simulink model "power_machines_Hatch"  (R2014a)
settings: Solver=ode23tb  SolverMode=SingleTasking  StartTime=0.0  StopTime=60  RelTol=1e-4
undefined symbols (not defined in the file or in its folder): A, B, C, Continuous, Dd, Ka, Ke, Kf, SeVe1, SeVe2, spsAC1AModel, Ta, Te, Tf, VAmax, VAmin, Ve0, Ve1, Ve2, Vfe0, VRmax, VRmin
undefined symbols (not defined in the file): Tb, Tc
libraries: sps_avr x19, powerlib x16, simulink_extras x4
(part 1 of 2)
Description:
  | Copyright 2008-2014 The MathWorks, Inc.
settings Model: FPTRunName=Active  ExtModeTrigMode=oneshot  ExtModeArmWhenConnect=off  ExtModeAutoUpdateStatusClock=off  Creator=MathWorks  LastModifiedBy=jdlara
settings SolverCC: ZeroCrossAlgorithm=Adaptive
settings DataIOCC: LimitDataPoints=off  SignalLoggingSaveFormat=ModelDataLogs  SignalLoggingName=sigsOut  OutputTimes=[0:1/20:10]
settings OptimizationCC: BlockReduction=off  BooleanDataType=off  ExpressionDepthLimit=2147483647  InitFltsAndDblsToZero=on  EfficientMapNaN2IntZero=off
settings DebuggingCC: UnderspecifiedInitializationDetection=Classic  CheckExecutionContextPreStartOutputMsg=on  CheckExecutionContextRuntimeOutputMsg=on  SignalResolutionControl=TryResolveAllWithWarning  IgnoredZcDiagnostic=none  SolverPrmCheckMsg=none  MultiTaskDSMMsg=warning  MultiTaskCondExecSysMsg=none  SigSpecEnsureSampleTimeMsg=none  FcnCallInpInsideContextMsg=UseLocalSettings  UnconnectedInputMsg=none  UnconnectedOutputMsg=none  UnconnectedLineMsg=none  StateNameClashWarn=warning
settings HardwareCC: ProdHWDeviceType=Specified  TargetUnknown=on
settings RTWCC: IncludeERTFirstTime=on
settings CodeAppCC: IgnoreCustomStorageClasses=off
settings GRTTargetCC: TargetFcnLib=ansi_tfl_tmw.mat  CombineOutputUpdateFcns=off  GRTInterface=on

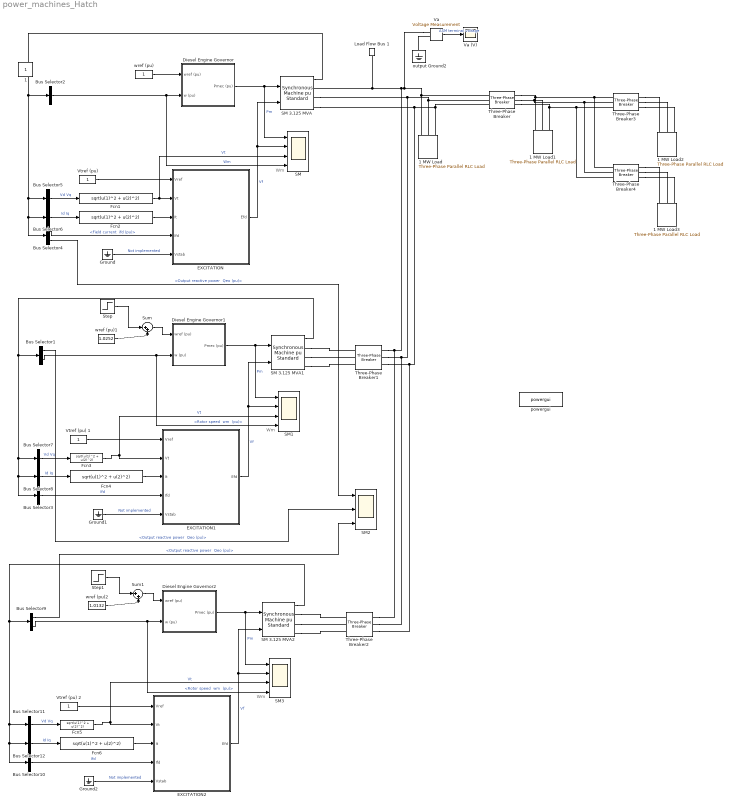
== system power_machines_Hatch ==
  note: Wm
  note: Wm
  note: Wm
  1 MW Load : powerlib/Elements/Three-Phase Parallel RLC Load  LConnTagsString=A|B|C  Configuration=Y (grounded)  NominalVoltage=2400  NominalFrequency=60  ActivePower=2.8e+006  InductivePower=8e5  CapacitivePower=0  Measurements=None  LoadType=constant Z
  1 MW Load1 : powerlib/Elements/Three-Phase Parallel RLC Load  LConnTagsString=A|B|C  Configuration=Y (grounded)  NominalVoltage=2400  NominalFrequency=60  ActivePower=1.5e+006  InductivePower=8e5  CapacitivePower=0  Measurements=None  LoadType=constant Z
  1 MW Load2 : powerlib/Elements/Three-Phase Parallel RLC Load  LConnTagsString=A|B|C  Configuration=Y (grounded)  NominalVoltage=2400  NominalFrequency=60  ActivePower=1.0e+006  InductivePower=8e5  CapacitivePower=0  Measurements=None  LoadType=constant Z
  1 MW Load3 : powerlib/Elements/Three-Phase Parallel RLC Load  LConnTagsString=A|B|C  Configuration=Y (grounded)  NominalVoltage=2400  NominalFrequency=60  ActivePower=1.1e+006  InductivePower=8e4  CapacitivePower=0  Measurements=None  LoadType=constant Z
  Bus Selector1 : BusSelector  OutputSignals="Output reactive power  Qeo (pu),Mechanical.Rotor speed  wm  (pu)"
  Bus Selector10 : BusSelector  OutputSignals="dq0 components.Field current  ifd (pu)"  OutputAsBus=on
  Bus Selector11 : BusSelector  OutputSignals="dq0 components.Stator voltage  vd (pu),dq0 components.Stator voltage  vq (pu)"  OutputAsBus=on
  Bus Selector12 : BusSelector  OutputSignals="dq0 components.Stator current  id (pu),dq0 components.Stator current  iq (pu)"  OutputAsBus=on
  Bus Selector2 : BusSelector  OutputSignals="Mechanical.Rotor speed  wm  (pu)"  OutputAsBus=on
  Bus Selector3 : BusSelector  OutputSignals="dq0 components.Field current  ifd (pu)"  OutputAsBus=on
  Bus Selector4 : BusSelector  OutputSignals="dq0 components.Field current  ifd (pu),Output reactive power  Qeo (pu)"
  Bus Selector5 : BusSelector  OutputSignals="dq0 components.Stator voltage  vd (pu),dq0 components.Stator voltage  vq (pu)"  OutputAsBus=on
  Bus Selector6 : BusSelector  OutputSignals="dq0 components.Stator current  id (pu),dq0 components.Stator current  iq (pu)"  OutputAsBus=on
  Bus Selector7 : BusSelector  OutputSignals="dq0 components.Stator voltage  vd (pu),dq0 components.Stator voltage  vq (pu)"  OutputAsBus=on
  Bus Selector8 : BusSelector  OutputSignals="dq0 components.Stator current  id (pu),dq0 components.Stator current  iq (pu)"  OutputAsBus=on
  Bus Selector9 : BusSelector  OutputSignals="Output reactive power  Qeo (pu),Mechanical.Rotor speed  wm  (pu)"
  Diesel Engine Governor : Subsystem  mask(Diesel Engine & Governor){K=40, Tr=[0.01 0.02 0.2], Ta=[0.25 0.009 0.0384], Tlim=[0 1.1], Td=0.024, Pm0=0.30302}
      mask prompts: K "Regulator gain K:"; Tr "Regulator time constants [T1 T2 T3 ] (s) :"; Ta "Actuator time constants [T4 T5 T6] (s) :"; Tlim "Torque limits [Tmin Tmax] (pu) :"; Td "Engine time delay Td (s) :"; Pm0 "Initial value of mechanical power  Pm0 (pu) :"
      mask help:
      | This block implements a diesel engine and governor system:
      | 1st and 2nd inputs: Desired and actual speed (pu)
      | Output: Diesel engine mechanical power.Motor inertia should be combined with generator.
      | Controller transfer function:
      |      Hc=K.(1+T3.s)/(1+T1.s+T1.T2.s^2)
      | Actuator transfer function :
      |      Ha= (1+T4.s) / [ (s (1+T5.s)(1+T6.s) ]
      | Motor :
      |      Time delay Td
      |
      | (See reference in Tutorial Session 5)
  Diesel Engine Governor1 : Subsystem  mask(Diesel Engine & Governor){K=40, Tr=[0.012 0.02 0.2], Ta=[0.25 0.009 0.0384], Tlim=[0 1.1], Td=0.024, Pm0=0.70051}
      mask prompts: K "Regulator gain K:"; Tr "Regulator time constants [T1 T2 T3 ] (s) :"; Ta "Actuator time constants [T4 T5 T6] (s) :"; Tlim "Torque limits [Tmin Tmax] (pu) :"; Td "Engine time delay Td (s) :"; Pm0 "Initial value of mechanical power  Pm0 (pu) :"
      mask help:
      | This block implements a diesel engine and governor system:
      | 1st and 2nd inputs: Desired and actual speed (pu)
      | Output: Diesel engine mechanical power.Motor inertia should be combined with generator.
      | Controller transfer function:
      |      Hc=K.(1+T3.s)/(1+T1.s+T1.T2.s^2)
      | Actuator transfer function :
      |      Ha= (1+T4.s) / [ (s (1+T5.s)(1+T6.s) ]
      | Motor :
      |      Time delay Td
      |
      | (See reference in Tutorial Session 5)
  Diesel Engine Governor2 : Subsystem  mask(Diesel Engine & Governor){K=40, Tr=[0.012 0.02 0.2], Ta=[0.25 0.009 0.0384], Tlim=[0 1.1], Td=0.024, Pm0=0.70051}
      mask prompts: K "Regulator gain K:"; Tr "Regulator time constants [T1 T2 T3 ] (s) :"; Ta "Actuator time constants [T4 T5 T6] (s) :"; Tlim "Torque limits [Tmin Tmax] (pu) :"; Td "Engine time delay Td (s) :"; Pm0 "Initial value of mechanical power  Pm0 (pu) :"
      mask help:
      | This block implements a diesel engine and governor system:
      | 1st and 2nd inputs: Desired and actual speed (pu)
      | Output: Diesel engine mechanical power.Motor inertia should be combined with generator.
      | Controller transfer function:
      |      Hc=K.(1+T3.s)/(1+T1.s+T1.T2.s^2)
      | Actuator transfer function :
      |      Ha= (1+T4.s) / [ (s (1+T5.s)(1+T6.s) ]
      | Motor :
      |      Time delay Td
      |
      | (See reference in Tutorial Session 5)
  EXCITATION : Subsystem  Variant=on  OverrideUsingVariant=Variant1
      settings: AttributesFormatString=%<BlockChoice>
  EXCITATION1 : Subsystem  Variant=on  OverrideUsingVariant=Variant1
      settings: AttributesFormatString=%<BlockChoice>
  EXCITATION2 : Subsystem  Variant=on  OverrideUsingVariant=Variant1
      settings: AttributesFormatString=%<BlockChoice>
  Fcn{1..6} (6 alike) : Fcn  Expr=sqrt(u(1)^2 + u(2)^2)
  Ground : Ground
  Ground1 : Ground
  Ground2 : Ground
  Load Flow Bus 1 : powerlib/Measurements/Load Flow Bus  LConnTagsString=a  ID=B2  Vbase=2.4e3  Vref=1  Vangle=0  VLF=1  angleLF=0
      settings: AttributesFormatString=%<ID>\n%<Vbase>V\n%<VLF>pu\n%<angleLF>deg.
  SM : Scope  NumInputPorts=4
      settings: TimeRange=45  YMin=0.3~-5~0~0.96  YMax=0.7000000000000001~10~1.5~1.04  SaveName=Pmec_SM1  DataFormat=Structure  Decimation=10
  SM 3.125 MVA : powerlib/Machines/Synchronous Machine pu Standard  PresetModel=No  MechanicalLoad=Mechanical power Pm  ShowDetailedParameters=on  RotorType=Salient-pole  Units=per unit standard parameters  MeasurementBus=off  NominalParameters="[ 3.125e6  2400  60]"  Reactances1=[ 31 32 33 34 35 36 37 ]  Reactances2=[ 1.56, 0.296, 0.177, 1.06, 0.177, 0.052 ]  dAxisTimeConstants=Short-circuit  qAxisTimeConstants=Open-circuit  TimeConstants1=[]  TimeConstants2=[]  TimeConstants3=[]  TimeConstants4=[]  TimeConstants5=[ 3.7, 0.05, 0.05 ]  TimeConstants6=[ 8.0, 0.03, 0.3371, 0.0295 ]  TimeConstants7=[0.024 0.006 0.006]  TimeConstants8=[]  StatorResistance=0.0036  Mechanical="[ 1.07  0 2]"  PolePairs=2  InitialConditions=[0 -78.3178 0.589753 0.589753 0.589753 -59.2242 -179.224 60.7758 1.84938]  SetSaturation=off  Saturation=[0.211 0.418 1.0 1.25 1.72 3.35 ;0.25 0.50 1.0 1.1 1.2 1.4]  LoadFlowParameters=[2 0 0 0]  TsPowergui=0  TsBlock=-1  IterativeModel=Forward Euler  BusType=swing  Pref=0  Qref=0  Qmin=-Inf  Qmax=Inf  PLF=0  QLF=0
      settings: AttributesFormatString=\n\n
  SM 3.125 MVA1 : powerlib/Machines/Synchronous Machine pu Standard  PresetModel=No  MechanicalLoad=Mechanical power Pm  ShowDetailedParameters=on  RotorType=Salient-pole  Units=per unit standard parameters  MeasurementBus=off  NominalParameters="[ 3.125e6  2400  60]"  Reactances1=[ 31 32 33 34 35 36 37 ]  Reactances2=[ 1.56, 0.296, 0.177, 1.06, 0.177, 0.052 ]  dAxisTimeConstants=Short-circuit  qAxisTimeConstants=Open-circuit  TimeConstants1=[]  TimeConstants2=[]  TimeConstants3=[]  TimeConstants4=[]  TimeConstants5=[ 3.7, 0.05, 0.05 ]  TimeConstants6=[ 8.0, 0.03, 0.3371, 0.0295 ]  TimeConstants7=[0.024 0.006 0.006]  TimeConstants8=[]  StatorResistance=0.0036  Mechanical="[ 1.07  0 2]"  PolePairs=2  InitialConditions=[0 -57.177 0.707662 0.707662 0.707662 -10.4209 -130.421 109.579 1.60133]  SetSaturation=off  Saturation=[0.211 0.418 1.0 1.25 1.72 3.35 ;0.25 0.50 1.0 1.1 1.2 1.4]  LoadFlowParameters=[4 0 0 0]  TsPowergui=0  TsBlock=-1  IterativeModel=Forward Euler  BusType=PQ  Pref=0.6987068134*3.125e6  Qref=0.4e6  Qmin=-Inf  Qmax=Inf  PLF=0  QLF=0
      settings: AttributesFormatString=\n\n
  SM 3.125 MVA2 : powerlib/Machines/Synchronous Machine pu Standard  PresetModel=No  MechanicalLoad=Mechanical power Pm  ShowDetailedParameters=on  RotorType=Salient-pole  Units=per unit standard parameters  MeasurementBus=off  NominalParameters="[ 3.125e6  2400  60]"  Reactances1=[ 31 32 33 34 35 36 37 ]  Reactances2=[ 1.56, 0.296, 0.177, 1.06, 0.177, 0.052 ]  dAxisTimeConstants=Short-circuit  qAxisTimeConstants=Open-circuit  TimeConstants1=[]  TimeConstants2=[]  TimeConstants3=[]  TimeConstants4=[]  TimeConstants5=[ 3.7, 0.05, 0.05 ]  TimeConstants6=[ 8.0, 0.03, 0.3371, 0.0295 ]  TimeConstants7=[0.024 0.006 0.006]  TimeConstants8=[]  StatorResistance=0.0036  Mechanical="[ 1.07  0 2]"  PolePairs=2  InitialConditions=[0 -57.177 0.707662 0.707662 0.707662 -10.4209 -130.421 109.579 1.60133]  SetSaturation=off  Saturation=[0.211 0.418 1.0 1.25 1.72 3.35 ;0.25 0.50 1.0 1.1 1.2 1.4]  LoadFlowParameters=[4 0 0 0]  TsPowergui=0  TsBlock=-1  IterativeModel=Forward Euler  BusType=PQ  Pref=0.6987068134*3.125e6  Qref=0.4e6  Qmin=-Inf  Qmax=Inf  PLF=0  QLF=0
      settings: AttributesFormatString=\n\n
  SM1 : Scope  NumInputPorts=4
      settings: TimeRange=4.8  YMin=0.7117940298507462~-5~1.0006~0.950028  YMax=0.7165940298507462~10~1.0016~1.05003  SaveName=Pmec_SM  DataFormat=Structure  Decimation=10
  SM2 : Scope  NumInputPorts=3
      settings: TimeRange=10  YMin=0~0~-5  YMax=1~1~5  SaveName=Pmec_SM2  DataFormat=Structure  Decimation=10
  SM3 : Scope  NumInputPorts=4
      settings: TimeRange=4.8  YMin=0.7117940298507462~-5~1.0006~0.950028  YMax=0.7165940298507462~10~1.0016~1.05003  SaveName=Pmec_SM3  DataFormat=Structure  Decimation=10
  Step : Step  Time=20  After=0.008  SampleTime=0
  Step1 : Step  Time=10  After=0.008  SampleTime=0
  Sum : Sum  Inputs=|++
  Sum1 : Sum  Inputs=|++
  Three-Phase Breaker : powerlib/Elements/Three-Phase Breaker  InitialState=closed  SwitchA=on  SwitchB=on  SwitchC=on  SwitchTimes="[92  170]"  External=off  BreakerResistance=0.01  SnubberResistance=1e6  SnubberCapacitance=inf  Measurements=None
  Three-Phase Breaker1 : powerlib/Elements/Three-Phase Breaker  InitialState=closed  SwitchA=on  SwitchB=on  SwitchC=on  SwitchTimes="[120  170]"  External=off  BreakerResistance=0.01  SnubberResistance=1e6  SnubberCapacitance=inf  Measurements=None
  Three-Phase Breaker2 : powerlib/Elements/Three-Phase Breaker  InitialState=closed  SwitchA=on  SwitchB=on  SwitchC=on  SwitchTimes="[120  170]"  External=off  BreakerResistance=0.01  SnubberResistance=1e6  SnubberCapacitance=inf  Measurements=None
  Three-Phase Breaker3 : powerlib/Elements/Three-Phase Breaker  InitialState=closed  SwitchA=on  SwitchB=on  SwitchC=on  SwitchTimes=[30 70]  External=off  BreakerResistance=0.01  SnubberResistance=1e6  SnubberCapacitance=inf  Measurements=None
  Three-Phase Breaker4 : powerlib/Elements/Three-Phase Breaker  InitialState=open  SwitchA=on  SwitchB=on  SwitchC=on  SwitchTimes=[40 70]  External=off  BreakerResistance=0.01  SnubberResistance=1e6  SnubberCapacitance=inf  Measurements=None
  Va : powerlib/Measurements/Voltage Measurement  Tag=PoWeRsYsTeMmEaSuReMeNt  PhasorSimulation=off  OutputType=Magnitude  PSBequivalent=0
  Va (V) : Scope
      settings: TickLabels=on  TimeRange=5  YMin=-3000  YMax=3000
  "Vtref (pu) " : Constant
  Vtref (pu) 1 : Constant
  Vtref (pu) 2 : Constant
  output Ground2 : powerlib/Elements/Ground  LConnTagsString=a
  powergui : powerlib/powergui  Priority=2  SimulationMode=Continuous  SolverType=Tustin  SampleTime=50e-6  frequency=60  SPID=off  DisableSnubberDevices=off  DisableRonSwitches=off  DisableVfSwitches=off  SwTol=0  Interpol=off  DisplayEquations=off  Ts=0  methode=off  frequencyindice=60  Pbase=1e6  ErrMax=0.0001  Iterations=50  UnitsV=kV  UnitsW=MW  FunctionMessages=off  echomessages=off  HookPort=off  EnableUseOfTLC=off  x0status=blocks  RestoreLinks=warning  ResistiveCurrentMeasurement=off  Frange=logspace(0,3,50)  Ylog=off  Xlog=off  ShowGrid=off  save=off  variable=ZData  structure=0  ZoomFFT=on  StartTime=0.0  cycles=2  DisplayStyle=off  fundamental=60  FreqAxis=off  MaxFrequency=1000  frequencyindicesteady=1  RmsSteady=1  display=off
  wref (pu) : Constant
  wref (pu)1 : Constant  Value=1.0252
  wref (pu)2 : Constant  Value=1.0132
  1 : Constant  IOType=siggen
  wires:
  Va/1 -> Va (V)/1  "ASM terminal voltage"
  Diesel Engine Governor/1(Pmec (pu)) -> SM/1, SM 3.125 MVA/1  "Pm"
  Fcn2/1 -> EXCITATION/3(It)
  Bus Selector4/1 -> EXCITATION/4(Ifd)  "<Field current  ifd (pu)>"
  Bus Selector6/1 -> Fcn2/1  "Id Iq"
  Ground/1 -> EXCITATION/5(Vstab)  "Not implemented"
  Bus Selector5/1 -> Fcn1/1  "Vd Vq"
  Bus Selector2/1 -> Diesel Engine Governor/2(w (pu)), SM/4  "Wm"
  Fcn1/1 -> EXCITATION/2(Vt), SM/3  "Vt"
  EXCITATION/1(Efd) -> SM 3.125 MVA/2, SM/2  "Vf"
  "Vtref (pu) "/1 -> EXCITATION/1(Vref)
  wref (pu)/1 -> Diesel Engine Governor/1(wref (pu))
  SM 3.125 MVA/1 -> Bus Selector2/1, Bus Selector5/1, Bus Selector6/1, Bus Selector4/1
  Diesel Engine Governor1/1(Pmec (pu)) -> SM1/1, SM 3.125 MVA1/1  "Pm"
  Fcn4/1 -> EXCITATION1/3(It)
  Bus Selector3/1 -> EXCITATION1/4(Ifd)  "Ifd"
  Bus Selector8/1 -> Fcn4/1  "Id Iq"
  Ground1/1 -> EXCITATION1/5(Vstab)  "Not implemented"
  Bus Selector7/1 -> Fcn3/1  "Vd Vq"
  Bus Selector1/2 -> Diesel Engine Governor1/2(w (pu)), SM1/4  "<Rotor speed  wm  (pu)>"
  Fcn3/1 -> EXCITATION1/2(Vt), SM1/3  "Vt"
  EXCITATION1/1(Efd) -> SM1/2, SM 3.125 MVA1/2  "Vf"
  Vtref (pu) 1/1 -> EXCITATION1/1(Vref)
  SM 3.125 MVA1/1 -> Bus Selector1/1, Bus Selector7/1, Bus Selector8/1, Bus Selector3/1
  Step/1 -> Sum/1
  wref (pu)1/1 -> Sum/2
  Sum/1 -> Diesel Engine Governor1/1(wref (pu))
  Bus Selector4/2 -> SM2/1  "<Output reactive power  Qeo (pu)>"
  Bus Selector1/1 -> SM2/2  "<Output reactive power  Qeo (pu)>"
  Diesel Engine Governor2/1(Pmec (pu)) -> SM3/1, SM 3.125 MVA2/1  "Pm"
  Fcn6/1 -> EXCITATION2/3(It)
  Bus Selector10/1 -> EXCITATION2/4(Ifd)  "Ifd"
  Bus Selector12/1 -> Fcn6/1  "Id Iq"
  Ground2/1 -> EXCITATION2/5(Vstab)  "Not implemented"
  Bus Selector11/1 -> Fcn5/1  "Vd Vq"
  Bus Selector9/2 -> Diesel Engine Governor2/2(w (pu)), SM3/4  "<Rotor speed  wm  (pu)>"
  Fcn5/1 -> EXCITATION2/2(Vt), SM3/3  "Vt"
  EXCITATION2/1(Efd) -> SM3/2, SM 3.125 MVA2/2  "Vf"
  Vtref (pu) 2/1 -> EXCITATION2/1(Vref)
  SM 3.125 MVA2/1 -> Bus Selector9/1, Bus Selector11/1, Bus Selector12/1, Bus Selector10/1
  Step1/1 -> Sum1/1
  wref (pu)2/1 -> Sum1/2
  Sum1/1 -> Diesel Engine Governor2/1(wref (pu))
  Bus Selector9/1 -> SM2/3  "<Output reactive power  Qeo (pu)>"
  connections:
  output Ground2/LConn1 -- Va/LConn2
  SM 3.125 MVA/RConn2 -- Three-Phase Breaker2/RConn2 -- Three-Phase Breaker1/RConn2 -- Three-Phase Breaker/LConn2 -- 1 MW Load/LConn2
  Va/LConn1 -- Three-Phase Breaker2/RConn1 -- Three-Phase Breaker1/RConn1 -- SM 3.125 MVA/RConn1 -- Load Flow Bus 1/LConn1 -- Three-Phase Breaker/LConn1 -- 1 MW Load/LConn1
  SM 3.125 MVA/RConn3 -- Three-Phase Breaker2/RConn3 -- Three-Phase Breaker1/RConn3 -- 1 MW Load/LConn3 -- Three-Phase Breaker/LConn3
  Three-Phase Breaker/RConn1 -- Three-Phase Breaker4/LConn1 -- Three-Phase Breaker3/LConn1 -- 1 MW Load1/LConn1
  Three-Phase Breaker/RConn2 -- Three-Phase Breaker4/LConn2 -- Three-Phase Breaker3/LConn2 -- 1 MW Load1/LConn2
  Three-Phase Breaker/RConn3 -- Three-Phase Breaker4/LConn3 -- Three-Phase Breaker3/LConn3 -- 1 MW Load1/LConn3
  SM 3.125 MVA1/RConn1 -- Three-Phase Breaker1/LConn1
  SM 3.125 MVA1/RConn2 -- Three-Phase Breaker1/LConn2
  SM 3.125 MVA1/RConn3 -- Three-Phase Breaker1/LConn3
  SM 3.125 MVA2/RConn1 -- Three-Phase Breaker2/LConn1
  SM 3.125 MVA2/RConn3 -- Three-Phase Breaker2/LConn3
  SM 3.125 MVA2/RConn2 -- Three-Phase Breaker2/LConn2
  Three-Phase Breaker3/RConn2 -- 1 MW Load2/LConn2
  Three-Phase Breaker3/RConn1 -- 1 MW Load2/LConn1
  Three-Phase Breaker3/RConn3 -- 1 MW Load2/LConn3
  Three-Phase Breaker4/RConn3 -- 1 MW Load3/LConn3
  Three-Phase Breaker4/RConn1 -- 1 MW Load3/LConn1
  Three-Phase Breaker4/RConn2 -- 1 MW Load3/LConn2

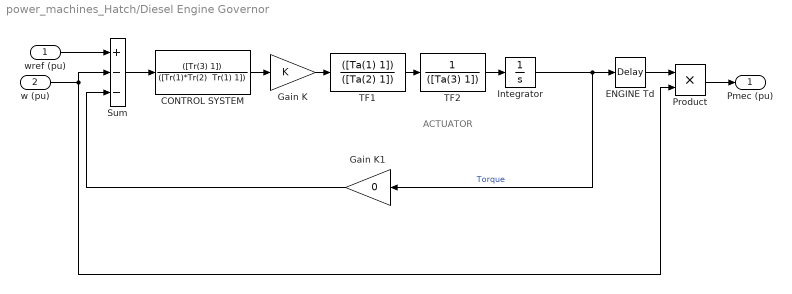
== system power_machines_Hatch/Diesel Engine Governor ==
  note: ACTUATOR
  wref (pu) : Inport
  w (pu) : Inport  Port=2
  CONTROL SYSTEM : TransferFcn  Numerator=([Tr(3) 1])  Denominator="([Tr(1)*Tr(2)  Tr(1) 1])"
  ENGINE Td : TransportDelay  DelayTime=Td  InitialOutput=Pm0
  Gain K : Gain  Gain=K  SaturateOnIntegerOverflow=on  OutDataTypeStr=Inherit: Same as input  ParamDataTypeStr=Inherit: Same as input
  Gain K1 : Gain  Gain=0  SaturateOnIntegerOverflow=on  OutDataTypeStr=Inherit: Same as input  ParamDataTypeStr=Inherit: Same as input
  Integrator : Integrator  InitialCondition=Pm0  LimitOutput=on  UpperSaturationLimit=Tlim(2)  LowerSaturationLimit=Tlim(1)
  Product : Product  SaturateOnIntegerOverflow=on  InputSameDT=on  OutDataTypeStr=Inherit: Same as first input
  Sum : Sum  Inputs=+--  SaturateOnIntegerOverflow=on  InputSameDT=on  OutDataTypeStr=Inherit: Same as first input
  TF1 : TransferFcn  Numerator=([Ta(1) 1])  Denominator=([Ta(2) 1])
  TF2 : TransferFcn  Numerator=1  Denominator=([Ta(3) 1])
  Pmec (pu) : Outport  InitialOutput=0
  wires:
  Integrator/1 -> Gain K1/1, ENGINE Td/1  "Torque"
  TF2/1 -> Integrator/1
  Product/1 -> Pmec (pu)/1
  wref (pu)/1 -> Sum/1
  ENGINE Td/1 -> Product/1
  w (pu)/1 -> Sum/2, Product/2
  TF1/1 -> TF2/1
  CONTROL SYSTEM/1 -> Gain K/1
  Sum/1 -> CONTROL SYSTEM/1
  Gain K/1 -> TF1/1
  Gain K1/1 -> Sum/3

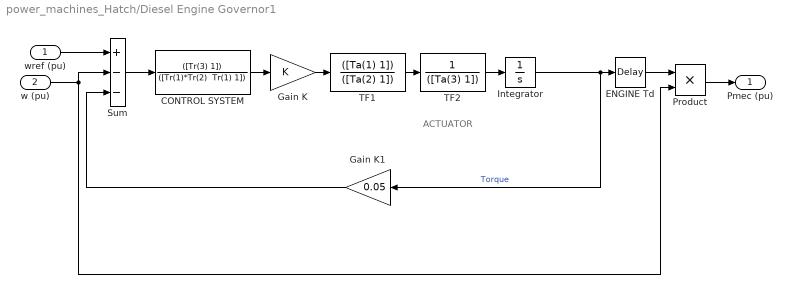
== system power_machines_Hatch/Diesel Engine Governor1 ==
  note: ACTUATOR
  wref (pu) : Inport
  w (pu) : Inport  Port=2
  CONTROL SYSTEM : TransferFcn  Numerator=([Tr(3) 1])  Denominator="([Tr(1)*Tr(2)  Tr(1) 1])"
  ENGINE Td : TransportDelay  DelayTime=Td  InitialOutput=Pm0
  Gain K : Gain  Gain=K  SaturateOnIntegerOverflow=on  OutDataTypeStr=Inherit: Same as input  ParamDataTypeStr=Inherit: Same as input
  Gain K1 : Gain  Gain=0.05  SaturateOnIntegerOverflow=on  OutDataTypeStr=Inherit: Same as input  ParamDataTypeStr=Inherit: Same as input
  Integrator : Integrator  InitialCondition=Pm0  LimitOutput=on  UpperSaturationLimit=Tlim(2)  LowerSaturationLimit=Tlim(1)
  Product : Product  SaturateOnIntegerOverflow=on  InputSameDT=on  OutDataTypeStr=Inherit: Same as first input
  Sum : Sum  Inputs=+--  SaturateOnIntegerOverflow=on  InputSameDT=on  OutDataTypeStr=Inherit: Same as first input
  TF1 : TransferFcn  Numerator=([Ta(1) 1])  Denominator=([Ta(2) 1])
  TF2 : TransferFcn  Numerator=1  Denominator=([Ta(3) 1])
  Pmec (pu) : Outport  InitialOutput=0
  wires:
  Integrator/1 -> Gain K1/1, ENGINE Td/1  "Torque"
  TF2/1 -> Integrator/1
  Product/1 -> Pmec (pu)/1
  wref (pu)/1 -> Sum/1
  ENGINE Td/1 -> Product/1
  w (pu)/1 -> Sum/2, Product/2
  TF1/1 -> TF2/1
  CONTROL SYSTEM/1 -> Gain K/1
  Sum/1 -> CONTROL SYSTEM/1
  Gain K/1 -> TF1/1
  Gain K1/1 -> Sum/3

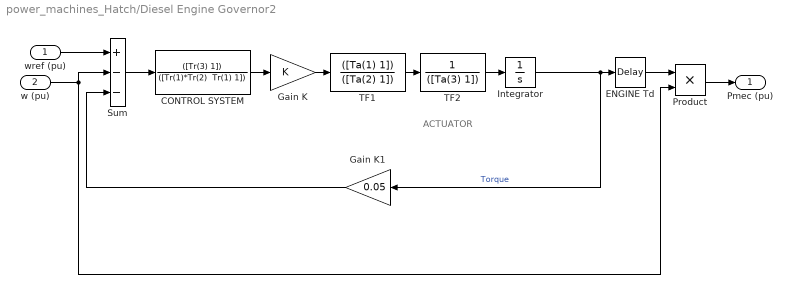
== system power_machines_Hatch/Diesel Engine Governor2 ==
  note: ACTUATOR
  wref (pu) : Inport
  w (pu) : Inport  Port=2
  CONTROL SYSTEM : TransferFcn  Numerator=([Tr(3) 1])  Denominator="([Tr(1)*Tr(2)  Tr(1) 1])"
  ENGINE Td : TransportDelay  DelayTime=Td  InitialOutput=Pm0
  Gain K : Gain  Gain=K  SaturateOnIntegerOverflow=on  OutDataTypeStr=Inherit: Same as input  ParamDataTypeStr=Inherit: Same as input
  Gain K1 : Gain  Gain=0.05  SaturateOnIntegerOverflow=on  OutDataTypeStr=Inherit: Same as input  ParamDataTypeStr=Inherit: Same as input
  Integrator : Integrator  InitialCondition=Pm0  LimitOutput=on  UpperSaturationLimit=Tlim(2)  LowerSaturationLimit=Tlim(1)
  Product : Product  SaturateOnIntegerOverflow=on  InputSameDT=on  OutDataTypeStr=Inherit: Same as first input
  Sum : Sum  Inputs=+--  SaturateOnIntegerOverflow=on  InputSameDT=on  OutDataTypeStr=Inherit: Same as first input
  TF1 : TransferFcn  Numerator=([Ta(1) 1])  Denominator=([Ta(2) 1])
  TF2 : TransferFcn  Numerator=1  Denominator=([Ta(3) 1])
  Pmec (pu) : Outport  InitialOutput=0
  wires:
  Integrator/1 -> Gain K1/1, ENGINE Td/1  "Torque"
  TF2/1 -> Integrator/1
  Product/1 -> Pmec (pu)/1
  wref (pu)/1 -> Sum/1
  ENGINE Td/1 -> Product/1
  w (pu)/1 -> Sum/2, Product/2
  TF1/1 -> TF2/1
  CONTROL SYSTEM/1 -> Gain K/1
  Sum/1 -> CONTROL SYSTEM/1
  Gain K/1 -> TF1/1
  Gain K1/1 -> Sum/3

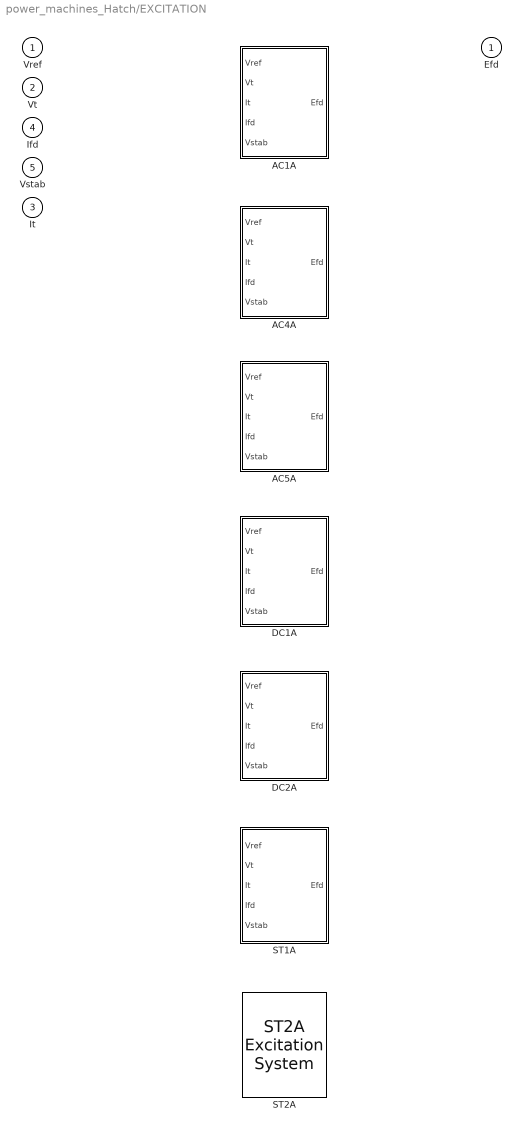
== system power_machines_Hatch/EXCITATION ==
  Vref : Inport
  Vt : Inport  Port=2
  It : Inport  Port=3
  Ifd : Inport  Port=4
  Vstab : Inport  Port=5
  AC1A : Subsystem  VariantControl=Variant1
  AC4A : Subsystem  VariantControl=Variant2
  AC5A : Subsystem  VariantControl=Variant3
  DC1A : Subsystem  VariantControl=Variant4
  DC2A : Subsystem  VariantControl=Variant5
  ST1A : Subsystem  VariantControl=Variant6
  ST2A : sps_avr/ST2A Excitation System  VariantControl=Variant7  Tr=20e-3  KaTa=[120 0.15]  VRminmax=[0 1.0]  KfTf=[0.05 1.0]  KeTe=[1.0 0.5]  KI=8.0  Kp=4.88  Xd=1.56  Kc=1.82  v0=[1,1.42734]  I0=0.2739  TsBlock=-2
  Efd : Outport

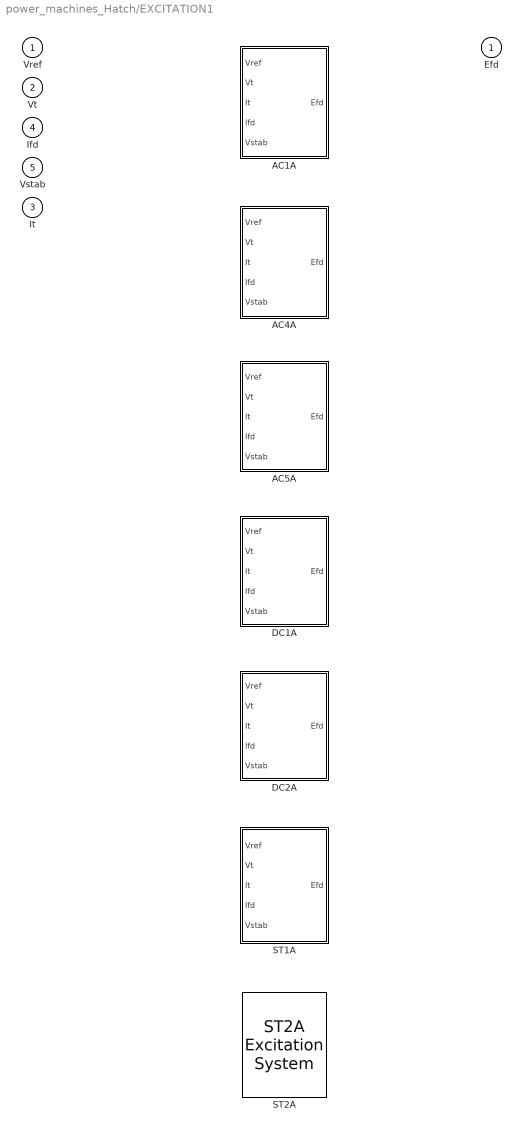
== system power_machines_Hatch/EXCITATION1 ==
  Vref : Inport
  Vt : Inport  Port=2
  It : Inport  Port=3
  Ifd : Inport  Port=4
  Vstab : Inport  Port=5
  AC1A : Subsystem  VariantControl=Variant1
  AC4A : Subsystem  VariantControl=Variant2
  AC5A : Subsystem  VariantControl=Variant3
  DC1A : Subsystem  VariantControl=Variant4
  DC2A : Subsystem  VariantControl=Variant5
  ST1A : Subsystem  VariantControl=Variant6
  ST2A : sps_avr/ST2A Excitation System  VariantControl=Variant7  Tr=20e-3  KaTa=[120 0.15]  VRminmax=[0 1.0]  KfTf=[0.05 1.0]  KeTe=[1.0 0.5]  KI=8.0  Kp=4.88  Xd=1.56  Kc=1.82  v0=[1,1.42734]  I0=0.2739  TsBlock=-2
  Efd : Outport

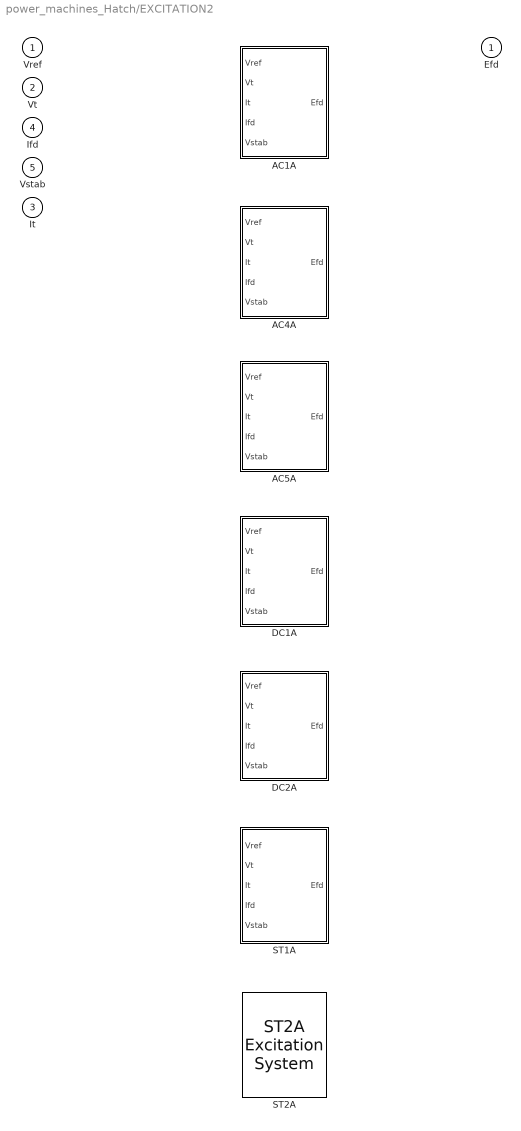
== system power_machines_Hatch/EXCITATION2 ==
  Vref : Inport
  Vt : Inport  Port=2
  It : Inport  Port=3
  Ifd : Inport  Port=4
  Vstab : Inport  Port=5
  AC1A : Subsystem  VariantControl=Variant1
  AC4A : Subsystem  VariantControl=Variant2
  AC5A : Subsystem  VariantControl=Variant3
  DC1A : Subsystem  VariantControl=Variant4
  DC2A : Subsystem  VariantControl=Variant5
  ST1A : Subsystem  VariantControl=Variant6
  ST2A : sps_avr/ST2A Excitation System  VariantControl=Variant7  Tr=20e-3  KaTa=[120 0.15]  VRminmax=[0 1.0]  KfTf=[0.05 1.0]  KeTe=[1.0 0.5]  KI=8.0  Kp=4.88  Xd=1.56  Kc=1.82  v0=[1,1.42734]  I0=0.2739  TsBlock=-2
  Efd : Outport

== system power_machines_Hatch/EXCITATION/AC1A ==
  Vref : Inport
  Vt : Inport  Port=2
  It : Inport  Port=3
  Ifd : Inport  Port=4
  Vstab : Inport  Port=5
  AC1A : sps_avr/AC1A Excitation System  Tr=20e-10  KaTa=[400 0.02]  VAminmax=[-14.5 14.5]  VRminmax=[-5.43 6.03]  KfTf=[0.03 1.0]  TbTc=[0 0]  KeTe=[1.0 0.80]  Ve12=[4.18 3.14]  SeVe12=[0.10 0.03]  Kd=0.38  Kc=0.20  v0=[1 1.8494]  TsBlock=-2
      link override Model/Continuous/Vfe0//Ka: Value=Vfe0/Ka
  term3 : Terminator
  Efd : Outport
  wires:
  It/1 -> term3/1
  AC1A/1 -> Efd/1
  Vstab/1 -> AC1A/4
  Ifd/1 -> AC1A/3
  Vt/1 -> AC1A/2
  Vref/1 -> AC1A/1

== system power_machines_Hatch/EXCITATION/AC4A ==
  Vref : Inport
  Vt : Inport  Port=2
  It : Inport  Port=3
  Ifd : Inport  Port=4
  Vstab : Inport  Port=5
  AC4A : sps_avr/AC4A Excitation System  Tr=20e-3  KaTa=[200 0.015]  VIminmax=[-10 10]  VRminmax=[-4.53 5.64]  TbTc=[10 1.0]  Kc=0  v0=[1,1.42734]  TsBlock=-2
  term3 : Terminator
  Efd : Outport
  wires:
  It/1 -> term3/1
  AC4A/1 -> Efd/1
  Vstab/1 -> AC4A/4
  Ifd/1 -> AC4A/3
  Vt/1 -> AC4A/2
  Vref/1 -> AC4A/1

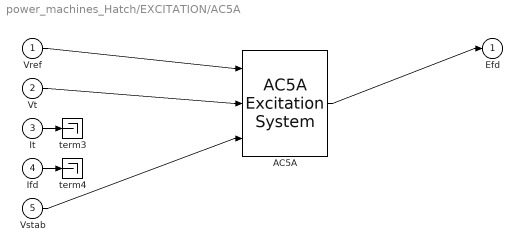
== system power_machines_Hatch/EXCITATION/AC5A ==
  Vref : Inport
  Vt : Inport  Port=2
  It : Inport  Port=3
  Ifd : Inport  Port=4
  Vstab : Inport  Port=5
  AC5A : sps_avr/AC5A Excitation System  Tr=20e-3  KaTa=[100 0.02]  VRminmax=[-7.3 7.3]  KfTf=[0.03 1 0 0]  KeTe=[1.0 0.02]  Efd12=[5.6 0.75*5.6]  SeEfd12=[0.86 0.5]  v0=[1,1.42734]  TsBlock=-2
  term3 : Terminator
  term4 : Terminator
  Efd : Outport
  wires:
  Ifd/1 -> term4/1
  It/1 -> term3/1
  AC5A/1 -> Efd/1
  Vstab/1 -> AC5A/3
  Vt/1 -> AC5A/2
  Vref/1 -> AC5A/1

== system power_machines_Hatch/EXCITATION/DC1A ==
  Vref : Inport
  Vt : Inport  Port=2
  It : Inport  Port=3
  Ifd : Inport  Port=4
  Vstab : Inport  Port=5
  DC1A : sps_avr/DC1A Excitation System  Tr=20e-3  KaTa=[46 0.06]  VRminmax=[-0.9 1.0]  KfTf=[0.05 1.5]  TbTc=[0 0]  KeTe=[0.05 0.46]  Efd12=[3.1 2.3]  SeEfd12=[0.33 0.10]  v0=[1,1.42734]  TsBlock=-2
  term3 : Terminator
  term4 : Terminator
  Efd : Outport
  wires:
  Ifd/1 -> term4/1
  It/1 -> term3/1
  DC1A/1 -> Efd/1
  Vstab/1 -> DC1A/3
  Vt/1 -> DC1A/2
  Vref/1 -> DC1A/1

== system power_machines_Hatch/EXCITATION/DC2A ==
  Vref : Inport
  Vt : Inport  Port=2
  It : Inport  Port=3
  Ifd : Inport  Port=4
  Vstab : Inport  Port=5
  DC2A : sps_avr/DC2A Excitation System  Tr=20e-3  KaTa=[46 0.06]  VRminmax=[-4.9 4.95]  KfTf=[0.05 1.5]  TbTc=[0 0]  KeTe=[0.05 0.46]  Efd12=[3.05 2.29]  SeEfd12=[0.279 0.117]  v0=[1,1.42734]  TsBlock=-2
  term3 : Terminator
  term4 : Terminator
  Efd : Outport
  wires:
  Ifd/1 -> term4/1
  It/1 -> term3/1
  DC2A/1 -> Efd/1
  Vstab/1 -> DC2A/3
  Vt/1 -> DC2A/2
  Vref/1 -> DC2A/1

== system power_machines_Hatch/EXCITATION/ST1A ==
  Vref : Inport
  Vt : Inport  Port=2
  It : Inport  Port=3
  Ifd : Inport  Port=4
  Vstab : Inport  Port=5
  ST1A : sps_avr/ST1A Excitation System  Tr=20e-3  KaTa=[210 0.001]  VIminmax=[-999 999]  VAminmax=[-999 999]  VRminmax=[-6.0 6.43]  KfTf=[0.001 1]  TbTc=[0 0 0 0]  KLR=1  ILR=2  Kc=0.038  v0=[1,1.42734]  TsBlock=-2
  term3 : Terminator
  Efd : Outport
  wires:
  It/1 -> term3/1
  ST1A/1 -> Efd/1
  Vstab/1 -> ST1A/4
  Ifd/1 -> ST1A/3
  Vt/1 -> ST1A/2
  Vref/1 -> ST1A/1

== system power_machines_Hatch/EXCITATION1/AC1A ==
  Vref : Inport
  Vt : Inport  Port=2
  It : Inport  Port=3
  Ifd : Inport  Port=4
  Vstab : Inport  Port=5
  AC1A : Subsystem  AncestorBlock=sps_avr/AC1A Excitation System  mask(AC1A Excitation System){Tr=20e-11, KaTa=[400 0.02], VAminmax=[-14.5 14.5], VRminmax=[-5.43 6.03], KfTf=[0.03 1.0], TbTc=[0 0], KeTe=[1.0 0.80], Ve12=[4.18 3.14], SeVe12=[0.10 0.03], Kd=0.38, Kc=0.20, v0=[1.0038 1.6013], TsBlock=-2}
      mask prompts: Tr "Low-pass filter time constant Tr(s):"; KaTa "Voltage regulator gain and time constant [Ka Ta(s)]:"; VAminmax "Voltage regulator internal limits [VAmin(pu) VAmax(pu)]:"; VRminmax "Voltage regulator output limits [VRmin(pu) VRmax(pu)]:"; KfTf "Damping filter gain and time constant [Kf Tf(s)]:"; TbTc "Transient gain reduction lead and lag time constants [Tb(s) Tc(s)]:"; KeTe "Exciter gain and time constant [Ke Te(s)]:"; Ve12 "Exciter alternator voltage values [Ve1(pu) Ve2(pu)]:"; SeVe12 "Exciter saturation function values [SeVe1(pu) SeVe2(pu)]:"; Kd "Demagnetizing factor Kd(pu):"; Kc "Rectifier loading factor Kc(pu):"; v0 "Initial values of terminal voltage and field voltage [Vt0(pu) Efd0(pu)]:"; TsBlock "Sample time:"
      mask help: Implements a synchronous machine voltage regulator and exciter based on the IEEE type AC1A excitation system model. The output is the field voltage to apply to the Vf input of a Synchronous Machine block. Inputs and output are in p.u.
      mask init:
      | block = gcb;
      | [Ts,BlockChoice,MaskType,Ka,Ta,Ke,Te,Kf,Tf,Tb,Tc,Ve1,Ve2,SeVe1,SeVe2,VRmin,VRmax,VAmin,VAmax,Ifd0,Ve0,Vfe0,Vt0,Efd0] = powericon('ExcitationSystemInit',block,TsBlock,KaTa,KeTe,KfTf,TbTc,Ve12,SeVe12,VRminmax,VAminmax,Kc,Kd,v0);
      | powericon('SetInternalModels','set',block,BlockChoice);
      mask Help: helpview(psbhelp);
      mask Display: color('blue');disp('AC1A')
  term3 : Terminator
  Efd : Outport
  wires:
  It/1 -> term3/1
  AC1A/1(Efd) -> Efd/1
  Vstab/1 -> AC1A/4(Vstab)
  Ifd/1 -> AC1A/3(Ifd)
  Vt/1 -> AC1A/2(Vt)
  Vref/1 -> AC1A/1(Vref)

== system power_machines_Hatch/EXCITATION1/AC4A ==
  Vref : Inport
  Vt : Inport  Port=2
  It : Inport  Port=3
  Ifd : Inport  Port=4
  Vstab : Inport  Port=5
  AC4A : sps_avr/AC4A Excitation System  Tr=20e-3  KaTa=[200 0.015]  VIminmax=[-10 10]  VRminmax=[-4.53 5.64]  TbTc=[10 1.0]  Kc=0  v0=[1,1.42734]  TsBlock=-2
  term3 : Terminator
  Efd : Outport
  wires:
  It/1 -> term3/1
  AC4A/1 -> Efd/1
  Vstab/1 -> AC4A/4
  Ifd/1 -> AC4A/3
  Vt/1 -> AC4A/2
  Vref/1 -> AC4A/1

== system power_machines_Hatch/EXCITATION1/AC5A ==
  Vref : Inport
  Vt : Inport  Port=2
  It : Inport  Port=3
  Ifd : Inport  Port=4
  Vstab : Inport  Port=5
  AC5A : sps_avr/AC5A Excitation System  Tr=20e-3  KaTa=[100 0.02]  VRminmax=[-7.3 7.3]  KfTf=[0.03 1 0 0]  KeTe=[1.0 0.02]  Efd12=[5.6 0.75*5.6]  SeEfd12=[0.86 0.5]  v0=[1,1.42734]  TsBlock=-2
  term3 : Terminator
  term4 : Terminator
  Efd : Outport
  wires:
  Ifd/1 -> term4/1
  It/1 -> term3/1
  AC5A/1 -> Efd/1
  Vstab/1 -> AC5A/3
  Vt/1 -> AC5A/2
  Vref/1 -> AC5A/1

== system power_machines_Hatch/EXCITATION1/DC1A ==
  Vref : Inport
  Vt : Inport  Port=2
  It : Inport  Port=3
  Ifd : Inport  Port=4
  Vstab : Inport  Port=5
  DC1A : sps_avr/DC1A Excitation System  Tr=20e-3  KaTa=[46 0.06]  VRminmax=[-0.9 1.0]  KfTf=[0.05 1.5]  TbTc=[0 0]  KeTe=[0.05 0.46]  Efd12=[3.1 2.3]  SeEfd12=[0.33 0.10]  v0=[1,1.42734]  TsBlock=-2
  term3 : Terminator
  term4 : Terminator
  Efd : Outport
  wires:
  Ifd/1 -> term4/1
  It/1 -> term3/1
  DC1A/1 -> Efd/1
  Vstab/1 -> DC1A/3
  Vt/1 -> DC1A/2
  Vref/1 -> DC1A/1

== system power_machines_Hatch/EXCITATION1/DC2A ==
  Vref : Inport
  Vt : Inport  Port=2
  It : Inport  Port=3
  Ifd : Inport  Port=4
  Vstab : Inport  Port=5
  DC2A : sps_avr/DC2A Excitation System  Tr=20e-3  KaTa=[46 0.06]  VRminmax=[-4.9 4.95]  KfTf=[0.05 1.5]  TbTc=[0 0]  KeTe=[0.05 0.46]  Efd12=[3.05 2.29]  SeEfd12=[0.279 0.117]  v0=[1,1.42734]  TsBlock=-2
  term3 : Terminator
  term4 : Terminator
  Efd : Outport
  wires:
  Ifd/1 -> term4/1
  It/1 -> term3/1
  DC2A/1 -> Efd/1
  Vstab/1 -> DC2A/3
  Vt/1 -> DC2A/2
  Vref/1 -> DC2A/1

== system power_machines_Hatch/EXCITATION1/ST1A ==
  Vref : Inport
  Vt : Inport  Port=2
  It : Inport  Port=3
  Ifd : Inport  Port=4
  Vstab : Inport  Port=5
  ST1A : sps_avr/ST1A Excitation System  Tr=20e-3  KaTa=[210 0.001]  VIminmax=[-999 999]  VAminmax=[-999 999]  VRminmax=[-6.0 6.43]  KfTf=[0.001 1]  TbTc=[0 0 0 0]  KLR=1  ILR=2  Kc=0.038  v0=[1,1.42734]  TsBlock=-2
  term3 : Terminator
  Efd : Outport
  wires:
  It/1 -> term3/1
  ST1A/1 -> Efd/1
  Vstab/1 -> ST1A/4
  Ifd/1 -> ST1A/3
  Vt/1 -> ST1A/2
  Vref/1 -> ST1A/1

== system power_machines_Hatch/EXCITATION2/AC1A ==
  Vref : Inport
  Vt : Inport  Port=2
  It : Inport  Port=3
  Ifd : Inport  Port=4
  Vstab : Inport  Port=5
  AC1A : Subsystem  AncestorBlock=sps_avr/AC1A Excitation System  mask(AC1A Excitation System){Tr=20e-11, KaTa=[400 0.02], VAminmax=[-14.5 14.5], VRminmax=[-5.43 6.03], KfTf=[0.03 1.0], TbTc=[0 0], KeTe=[1.0 0.80], Ve12=[4.18 3.14], SeVe12=[0.10 0.03], Kd=0.38, Kc=0.20, v0=[1.0038 1.6013], TsBlock=-2}
      mask prompts: Tr "Low-pass filter time constant Tr(s):"; KaTa "Voltage regulator gain and time constant [Ka Ta(s)]:"; VAminmax "Voltage regulator internal limits [VAmin(pu) VAmax(pu)]:"; VRminmax "Voltage regulator output limits [VRmin(pu) VRmax(pu)]:"; KfTf "Damping filter gain and time constant [Kf Tf(s)]:"; TbTc "Transient gain reduction lead and lag time constants [Tb(s) Tc(s)]:"; KeTe "Exciter gain and time constant [Ke Te(s)]:"; Ve12 "Exciter alternator voltage values [Ve1(pu) Ve2(pu)]:"; SeVe12 "Exciter saturation function values [SeVe1(pu) SeVe2(pu)]:"; Kd "Demagnetizing factor Kd(pu):"; Kc "Rectifier loading factor Kc(pu):"; v0 "Initial values of terminal voltage and field voltage [Vt0(pu) Efd0(pu)]:"; TsBlock "Sample time:"
      mask help: Implements a synchronous machine voltage regulator and exciter based on the IEEE type AC1A excitation system model. The output is the field voltage to apply to the Vf input of a Synchronous Machine block. Inputs and output are in p.u.
      mask init: same as power_machines_Hatch/EXCITATION1/AC1A/AC1A
      mask Help: helpview(psbhelp);
      mask Display: color('blue');disp('AC1A')
  term3 : Terminator
  Efd : Outport
  wires:
  It/1 -> term3/1
  AC1A/1(Efd) -> Efd/1
  Vstab/1 -> AC1A/4(Vstab)
  Ifd/1 -> AC1A/3(Ifd)
  Vt/1 -> AC1A/2(Vt)
  Vref/1 -> AC1A/1(Vref)

== system power_machines_Hatch/EXCITATION2/AC4A ==
  Vref : Inport
  Vt : Inport  Port=2
  It : Inport  Port=3
  Ifd : Inport  Port=4
  Vstab : Inport  Port=5
  AC4A : sps_avr/AC4A Excitation System  Tr=20e-3  KaTa=[200 0.015]  VIminmax=[-10 10]  VRminmax=[-4.53 5.64]  TbTc=[10 1.0]  Kc=0  v0=[1,1.42734]  TsBlock=-2
  term3 : Terminator
  Efd : Outport
  wires:
  It/1 -> term3/1
  AC4A/1 -> Efd/1
  Vstab/1 -> AC4A/4
  Ifd/1 -> AC4A/3
  Vt/1 -> AC4A/2
  Vref/1 -> AC4A/1

== system power_machines_Hatch/EXCITATION2/AC5A ==
  Vref : Inport
  Vt : Inport  Port=2
  It : Inport  Port=3
  Ifd : Inport  Port=4
  Vstab : Inport  Port=5
  AC5A : sps_avr/AC5A Excitation System  Tr=20e-3  KaTa=[100 0.02]  VRminmax=[-7.3 7.3]  KfTf=[0.03 1 0 0]  KeTe=[1.0 0.02]  Efd12=[5.6 0.75*5.6]  SeEfd12=[0.86 0.5]  v0=[1,1.42734]  TsBlock=-2
  term3 : Terminator
  term4 : Terminator
  Efd : Outport
  wires:
  Ifd/1 -> term4/1
  It/1 -> term3/1
  AC5A/1 -> Efd/1
  Vstab/1 -> AC5A/3
  Vt/1 -> AC5A/2
  Vref/1 -> AC5A/1

== system power_machines_Hatch/EXCITATION2/DC1A ==
  Vref : Inport
  Vt : Inport  Port=2
  It : Inport  Port=3
  Ifd : Inport  Port=4
  Vstab : Inport  Port=5
  DC1A : sps_avr/DC1A Excitation System  Tr=20e-3  KaTa=[46 0.06]  VRminmax=[-0.9 1.0]  KfTf=[0.05 1.5]  TbTc=[0 0]  KeTe=[0.05 0.46]  Efd12=[3.1 2.3]  SeEfd12=[0.33 0.10]  v0=[1,1.42734]  TsBlock=-2
  term3 : Terminator
  term4 : Terminator
  Efd : Outport
  wires:
  Ifd/1 -> term4/1
  It/1 -> term3/1
  DC1A/1 -> Efd/1
  Vstab/1 -> DC1A/3
  Vt/1 -> DC1A/2
  Vref/1 -> DC1A/1

== system power_machines_Hatch/EXCITATION2/DC2A ==
  Vref : Inport
  Vt : Inport  Port=2
  It : Inport  Port=3
  Ifd : Inport  Port=4
  Vstab : Inport  Port=5
  DC2A : sps_avr/DC2A Excitation System  Tr=20e-3  KaTa=[46 0.06]  VRminmax=[-4.9 4.95]  KfTf=[0.05 1.5]  TbTc=[0 0]  KeTe=[0.05 0.46]  Efd12=[3.05 2.29]  SeEfd12=[0.279 0.117]  v0=[1,1.42734]  TsBlock=-2
  term3 : Terminator
  term4 : Terminator
  Efd : Outport
  wires:
  Ifd/1 -> term4/1
  It/1 -> term3/1
  DC2A/1 -> Efd/1
  Vstab/1 -> DC2A/3
  Vt/1 -> DC2A/2
  Vref/1 -> DC2A/1

== system power_machines_Hatch/EXCITATION2/ST1A ==
  Vref : Inport
  Vt : Inport  Port=2
  It : Inport  Port=3
  Ifd : Inport  Port=4
  Vstab : Inport  Port=5
  ST1A : sps_avr/ST1A Excitation System  Tr=20e-3  KaTa=[210 0.001]  VIminmax=[-999 999]  VAminmax=[-999 999]  VRminmax=[-6.0 6.43]  KfTf=[0.001 1]  TbTc=[0 0 0 0]  KLR=1  ILR=2  Kc=0.038  v0=[1,1.42734]  TsBlock=-2
  term3 : Terminator
  Efd : Outport
  wires:
  It/1 -> term3/1
  ST1A/1 -> Efd/1
  Vstab/1 -> ST1A/4
  Ifd/1 -> ST1A/3
  Vt/1 -> ST1A/2
  Vref/1 -> ST1A/1

== system power_machines_Hatch/EXCITATION1/AC1A/AC1A ==
  Vref : Inport
  Vt : Inport  Port=2
  Ifd : Inport  Port=3
  Vstab : Inport  Port=4
  Model : Subsystem  BlockChoice=Continuous
      link override Continuous/Vfe0//Ka: Value=Vfe0/Ka
      settings: AttributesFormatString=%<BlockChoice>  TemplateBlock=spsAC1AModel/Model  MemberBlocks=Continuous,Discrete
  Efd : Outport
  wires:
  Model/1(Efd) -> Efd/1
  Vstab/1 -> Model/4(Vstab)
  Ifd/1 -> Model/3(Ifd)
  Vt/1 -> Model/2(Vt)
  Vref/1 -> Model/1(Vref)

== system power_machines_Hatch/EXCITATION2/AC1A/AC1A ==
  Vref : Inport
  Vt : Inport  Port=2
  Ifd : Inport  Port=3
  Vstab : Inport  Port=4
  Model : Subsystem  BlockChoice=Continuous
      link override Continuous/Vfe0//Ka: Value=Vfe0/Ka
      settings: AttributesFormatString=%<BlockChoice>  TemplateBlock=spsAC1AModel/Model  MemberBlocks=Continuous,Discrete
  Efd : Outport
  wires:
  Model/1(Efd) -> Efd/1
  Vstab/1 -> Model/4(Vstab)
  Ifd/1 -> Model/3(Ifd)
  Vt/1 -> Model/2(Vt)
  Vref/1 -> Model/1(Vref)

== system power_machines_Hatch/EXCITATION1/AC1A/AC1A/Model ==
  Vref : Inport
  Vt : Inport  Port=2
  Ifd : Inport  Port=3
  Vstab : Inport  Port=4
  Continuous : Subsystem  AncestorBlock=spsAC1AModel/Continuous  mask(Excitation System){}
  Efd : Outport
  wires:
  Vref/1 -> Continuous/1(Vref)
  Vt/1 -> Continuous/2(Vt)
  Ifd/1 -> Continuous/3(Ifd)
  Vstab/1 -> Continuous/4(Vstab)
  Continuous/1(Efd) -> Efd/1

== system power_machines_Hatch/EXCITATION2/AC1A/AC1A/Model ==
  Vref : Inport
  Vt : Inport  Port=2
  Ifd : Inport  Port=3
  Vstab : Inport  Port=4
  Continuous : Subsystem  AncestorBlock=spsAC1AModel/Continuous  mask(Excitation System){}
  Efd : Outport
  wires:
  Vref/1 -> Continuous/1(Vref)
  Vt/1 -> Continuous/2(Vt)
  Ifd/1 -> Continuous/3(Ifd)
  Vstab/1 -> Continuous/4(Vstab)
  Continuous/1(Efd) -> Efd/1

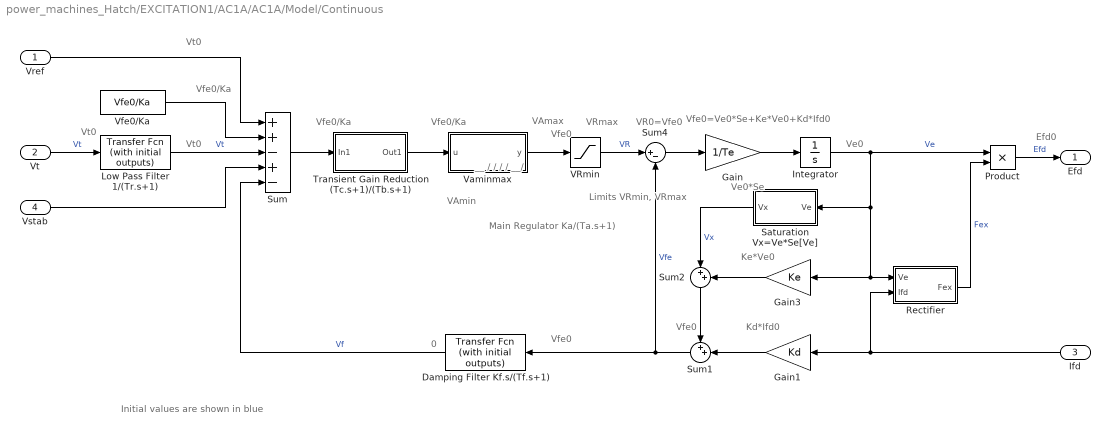
== system power_machines_Hatch/EXCITATION1/AC1A/AC1A/Model/Continuous ==
  note: VRmax
  note: VAmax
  note: VAmin
  note: __
      |              /
      |           /
      |         /
      |       /
      | __/
  note: Main Regulator
      | Ka/(Ta.s+1)
  note: Initial values are shown in blue
  note: Vfe0/Ka
  note: Vfe0/Ka
  note: Vfe0
  note: Ve0
  note: Vfe0
  note: Ve0*Se
  note: Ke*Ve0
  note: Kd*Ifd0
  note: Efd0
  note: 0
  note: Limits VRmin, VRmax
  note: Vt0
  note: Vt0
  note: Vfe0/Ka
  note: VR0=Vfe0
  note: Vfe0=Ve0*Se+Ke*Ve0+Kd*Ifd0
  note: Vfe0
  note: Vt0
  Vref : Inport
  Vt : Inport  Port=2
  Ifd : Inport  Port=3
  Vstab : Inport  Port=4
  Damping Filter Kf.s/(Tf.s+1) : simulink_extras/Additional Linear/Transfer Fcn (with initial outputs)  N=[Kf 0]  D=[Tf 1]  Y0=0  U0=Vfe0
  Gain : Gain  Gain=1/Te  SaturateOnIntegerOverflow=on  OutDataTypeStr=Inherit: Same as input  ParamDataTypeStr=Inherit: Same as input
  Gain1 : Gain  Gain=Kd  SaturateOnIntegerOverflow=on  OutDataTypeStr=Inherit: Same as input  ParamDataTypeStr=Inherit: Same as input
  Gain3 : Gain  Gain=Ke  SaturateOnIntegerOverflow=on  OutDataTypeStr=Inherit: Same as input  ParamDataTypeStr=Inherit: Same as input
  Integrator : Integrator  InitialCondition=Ve0  LimitOutput=on  LowerSaturationLimit=0
  Low Pass Filter 1/(Tr.s+1) : simulink_extras/Additional Linear/Transfer Fcn (with initial outputs)  N=1  D=[Tr 1]  Y0=Vt0  U0=Vt0
  Product : Product  SaturateOnIntegerOverflow=on  RndMeth=Zero  InputSameDT=on  OutDataTypeStr=Inherit: Same as first input
  Rectifier : Subsystem  mask{Kc=Kc}
      mask prompts: Kc "Rectifier loading factor Kc(pu):"
  Saturation Vx=Ve*Se[Ve] : Subsystem  mask{Ve12=[Ve1 Ve2], SeVe12=[SeVe1 SeVe2]}
      mask prompts: Ve12 "Exciter alternator voltage values [Ve1(pu) Ve2(pu)]:"; SeVe12 "Exciter saturation function values [SeVe1(pu) SeVe2(pu)]:"
      mask init:
      | Ve1=Ve12(1);Ve2=Ve12(2);
      | SeVe1=SeVe12(1);SeVe2=SeVe12(2);
  Sum : Sum  Inputs=++-+-  SaturateOnIntegerOverflow=on  InputSameDT=on  OutDataTypeStr=Inherit: Same as first input
  Sum1 : Sum  Inputs=++|  SaturateOnIntegerOverflow=on  InputSameDT=on  OutDataTypeStr=Inherit: Same as first input
  Sum2 : Sum  Inputs=|++  SaturateOnIntegerOverflow=on  InputSameDT=on  OutDataTypeStr=Inherit: Same as first input
  Sum4 : Sum  Inputs=|+-  SaturateOnIntegerOverflow=on  InputSameDT=on  OutDataTypeStr=Inherit: Same as first input
  Transient Gain Reduction (Tc.s+1)/(Tb.s+1) : Subsystem  mask(Transfer Function with Initial Outputs){N=[Tc 1], D=[Tb 1], Y0=Vfe0/Ka, U0=Vfe0/Ka}
      mask prompts: N "Numerator:"; D "Denominator:"; Y0 "Initial output:"; U0 "Initial input:"
      mask help: Vector expressions for numerator, and denominator. Coefficients are in descending powers of s.
      mask init:
      | [A,B,C,Dd]=tf2ss(N,D);if (isempty(Y0));[m,n]=size(A);X0=zeros(1,m); end; if (isempty(U0));[m,p]=size(B);U0=zeros(1,p);end;
      |  if isempty(A),  X0=[]; else ,X0=getxo(A,B,C,Dd,U0,Y0,0); end
      mask Help: Specify the initial output for the transfer function.  An optimization routine attempts to determine the appropriate initial states so that the specified initial output is achieved.  For more details, see the m-file getxo.m
      mask Display: dpoly(N,D,'s')
  VRmin : Saturate  UpperLimit=VRmax  LowerLimit=VRmin
  Vaminmax : Subsystem  mask{Ka=Ka, Ta=Ta, VAminmax=[VAmin VAmax], X0=Vfe0}
      mask prompts: Ka "Voltage regulator gain Ka:"; Ta "Voltage regulator time constant Ta(s):"; VAminmax "Voltage regulator internal limits [VAmin(pu) VAmax(pu)]:"; X0 "Initial conditions:"
      mask init:
      | VAmin=VAminmax(1);VAmax=VAminmax(2);
      mask Display: dpoly([Ka],[Ta 1],'s')
  Vfe0/Ka : Constant  Value=Vfe0/Ka
  Efd : Outport
  wires:
  VRmin/1 -> Sum4/1  "VR"
  Sum1/1 -> Sum4/2, Damping Filter Kf.s/(Tf.s+1)/1  "Vfe"
  Gain/1 -> Integrator/1
  Integrator/1 -> Product/1, Rectifier/1(Ve), Gain3/1, Saturation Vx=Ve*Se[Ve]/1(Ve)  "Ve"
  Sum2/1 -> Sum1/1
  Gain1/1 -> Sum1/2
  Gain3/1 -> Sum2/2
  Ifd/1 -> Rectifier/2(Ifd), Gain1/1
  Saturation Vx=Ve*Se[Ve]/1(Vx) -> Sum2/1  "Vx"
  Rectifier/1(Fex) -> Product/2  "Fex"
  Product/1 -> Efd/1  "Efd"
  Sum4/1 -> Gain/1
  Vaminmax/1(y) -> VRmin/1
  Sum/1 -> Transient Gain Reduction (Tc.s+1)/(Tb.s+1)/1(In1)
  Transient Gain Reduction (Tc.s+1)/(Tb.s+1)/1(Out1) -> Vaminmax/1(u)
  Vt/1 -> Low Pass Filter 1/(Tr.s+1)/1  "Vt"
  Vref/1 -> Sum/1
  Vfe0/Ka/1 -> Sum/2
  Low Pass Filter 1/(Tr.s+1)/1 -> Sum/3  "Vt"
  Damping Filter Kf.s/(Tf.s+1)/1 -> Sum/5  "Vf"
  Vstab/1 -> Sum/4

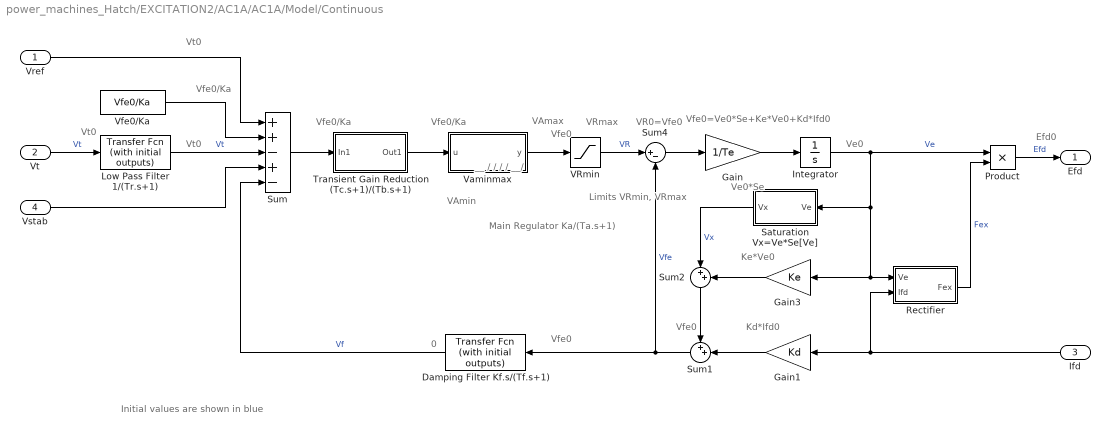
== system power_machines_Hatch/EXCITATION2/AC1A/AC1A/Model/Continuous ==
  note: VRmax
  note: VAmax
  note: VAmin
  note: __
      |              /
      |           /
      |         /
      |       /
      | __/
  note: Main Regulator
      | Ka/(Ta.s+1)
  note: Initial values are shown in blue
  note: Vfe0/Ka
  note: Vfe0/Ka
  note: Vfe0
  note: Ve0
  note: Vfe0
  note: Ve0*Se
  note: Ke*Ve0
  note: Kd*Ifd0
  note: Efd0
  note: 0
  note: Limits VRmin, VRmax
  note: Vt0
  note: Vt0
  note: Vfe0/Ka
  note: VR0=Vfe0
  note: Vfe0=Ve0*Se+Ke*Ve0+Kd*Ifd0
  note: Vfe0
  note: Vt0
  Vref : Inport
  Vt : Inport  Port=2
  Ifd : Inport  Port=3
  Vstab : Inport  Port=4
  Damping Filter Kf.s/(Tf.s+1) : simulink_extras/Additional Linear/Transfer Fcn (with initial outputs)  N=[Kf 0]  D=[Tf 1]  Y0=0  U0=Vfe0
  Gain : Gain  Gain=1/Te  SaturateOnIntegerOverflow=on  OutDataTypeStr=Inherit: Same as input  ParamDataTypeStr=Inherit: Same as input
  Gain1 : Gain  Gain=Kd  SaturateOnIntegerOverflow=on  OutDataTypeStr=Inherit: Same as input  ParamDataTypeStr=Inherit: Same as input
  Gain3 : Gain  Gain=Ke  SaturateOnIntegerOverflow=on  OutDataTypeStr=Inherit: Same as input  ParamDataTypeStr=Inherit: Same as input
  Integrator : Integrator  InitialCondition=Ve0  LimitOutput=on  LowerSaturationLimit=0
  Low Pass Filter 1/(Tr.s+1) : simulink_extras/Additional Linear/Transfer Fcn (with initial outputs)  N=1  D=[Tr 1]  Y0=Vt0  U0=Vt0
  Product : Product  SaturateOnIntegerOverflow=on  RndMeth=Zero  InputSameDT=on  OutDataTypeStr=Inherit: Same as first input
  Rectifier : Subsystem  mask{Kc=Kc}
      mask prompts: Kc "Rectifier loading factor Kc(pu):"
  Saturation Vx=Ve*Se[Ve] : Subsystem  mask{Ve12=[Ve1 Ve2], SeVe12=[SeVe1 SeVe2]}
      mask prompts: Ve12 "Exciter alternator voltage values [Ve1(pu) Ve2(pu)]:"; SeVe12 "Exciter saturation function values [SeVe1(pu) SeVe2(pu)]:"
      mask init:
      | Ve1=Ve12(1);Ve2=Ve12(2);
      | SeVe1=SeVe12(1);SeVe2=SeVe12(2);
  Sum : Sum  Inputs=++-+-  SaturateOnIntegerOverflow=on  InputSameDT=on  OutDataTypeStr=Inherit: Same as first input
  Sum1 : Sum  Inputs=++|  SaturateOnIntegerOverflow=on  InputSameDT=on  OutDataTypeStr=Inherit: Same as first input
  Sum2 : Sum  Inputs=|++  SaturateOnIntegerOverflow=on  InputSameDT=on  OutDataTypeStr=Inherit: Same as first input
  Sum4 : Sum  Inputs=|+-  SaturateOnIntegerOverflow=on  InputSameDT=on  OutDataTypeStr=Inherit: Same as first input
  Transient Gain Reduction (Tc.s+1)/(Tb.s+1) : Subsystem  mask(Transfer Function with Initial Outputs){N=[Tc 1], D=[Tb 1], Y0=Vfe0/Ka, U0=Vfe0/Ka}
      mask prompts: N "Numerator:"; D "Denominator:"; Y0 "Initial output:"; U0 "Initial input:"
      mask help: Vector expressions for numerator, and denominator. Coefficients are in descending powers of s.
      mask init:
      | [A,B,C,Dd]=tf2ss(N,D);if (isempty(Y0));[m,n]=size(A);X0=zeros(1,m); end; if (isempty(U0));[m,p]=size(B);U0=zeros(1,p);end;
      |  if isempty(A),  X0=[]; else ,X0=getxo(A,B,C,Dd,U0,Y0,0); end
      mask Help: Specify the initial output for the transfer function.  An optimization routine attempts to determine the appropriate initial states so that the specified initial output is achieved.  For more details, see the m-file getxo.m
      mask Display: dpoly(N,D,'s')
  VRmin : Saturate  UpperLimit=VRmax  LowerLimit=VRmin
  Vaminmax : Subsystem  mask{Ka=Ka, Ta=Ta, VAminmax=[VAmin VAmax], X0=Vfe0}
      mask prompts: Ka "Voltage regulator gain Ka:"; Ta "Voltage regulator time constant Ta(s):"; VAminmax "Voltage regulator internal limits [VAmin(pu) VAmax(pu)]:"; X0 "Initial conditions:"
      mask init:
      | VAmin=VAminmax(1);VAmax=VAminmax(2);
      mask Display: dpoly([Ka],[Ta 1],'s')
  Vfe0/Ka : Constant  Value=Vfe0/Ka
  Efd : Outport
  wires:
  VRmin/1 -> Sum4/1  "VR"
  Sum1/1 -> Sum4/2, Damping Filter Kf.s/(Tf.s+1)/1  "Vfe"
  Gain/1 -> Integrator/1
  Integrator/1 -> Product/1, Rectifier/1(Ve), Gain3/1, Saturation Vx=Ve*Se[Ve]/1(Ve)  "Ve"
  Sum2/1 -> Sum1/1
  Gain1/1 -> Sum1/2
  Gain3/1 -> Sum2/2
  Ifd/1 -> Rectifier/2(Ifd), Gain1/1
  Saturation Vx=Ve*Se[Ve]/1(Vx) -> Sum2/1  "Vx"
  Rectifier/1(Fex) -> Product/2  "Fex"
  Product/1 -> Efd/1  "Efd"
  Sum4/1 -> Gain/1
  Vaminmax/1(y) -> VRmin/1
  Sum/1 -> Transient Gain Reduction (Tc.s+1)/(Tb.s+1)/1(In1)
  Transient Gain Reduction (Tc.s+1)/(Tb.s+1)/1(Out1) -> Vaminmax/1(u)
  Vt/1 -> Low Pass Filter 1/(Tr.s+1)/1  "Vt"
  Vref/1 -> Sum/1
  Vfe0/Ka/1 -> Sum/2
  Low Pass Filter 1/(Tr.s+1)/1 -> Sum/3  "Vt"
  Damping Filter Kf.s/(Tf.s+1)/1 -> Sum/5  "Vf"
  Vstab/1 -> Sum/4

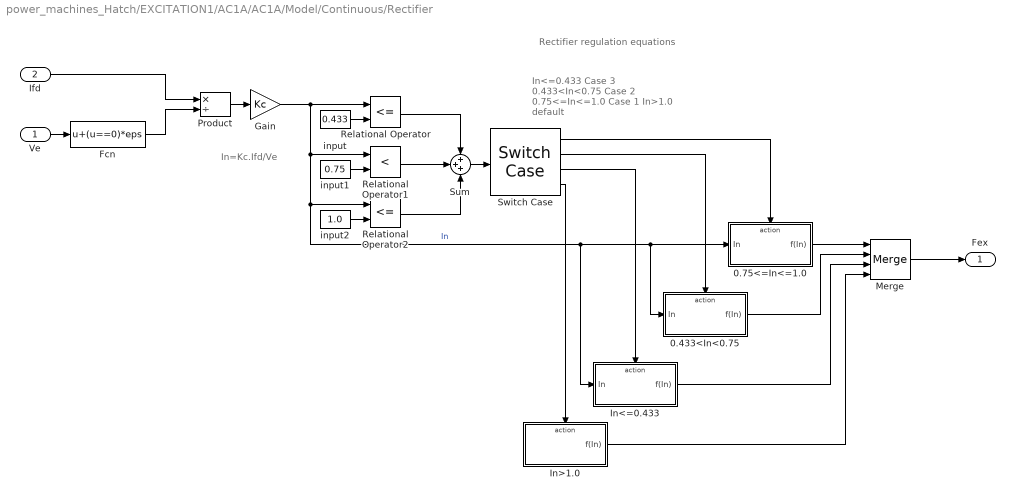
== system power_machines_Hatch/EXCITATION1/AC1A/AC1A/Model/Continuous/Rectifier ==
  note: In<=0.433        Case 3
      | 0.433<In<0.75 Case 2
      | 0.75<=In<=1.0 Case 1
      | In>1.0               default
  note: Rectifier regulation equations
  note: In=Kc.Ifd/Ve
  Ve : Inport
  Ifd : Inport  Port=2
  0.433<In<0.75 : Subsystem  TreatAsAtomicUnit=on
  0.75<=In<=1.0 : Subsystem  TreatAsAtomicUnit=on
  Fcn : Fcn  Expr=u+(u==0)*eps
  Gain : Gain  Gain=Kc  SaturateOnIntegerOverflow=on  OutDataTypeStr=Inherit: Same as input  ParamDataTypeStr=Inherit: Same as input
  In<=0.433 : Subsystem  TreatAsAtomicUnit=on
  In>1.0 : Subsystem  TreatAsAtomicUnit=on
  Merge : Merge  Inputs=4
  Product : Product  Inputs=*/  SaturateOnIntegerOverflow=on  RndMeth=Zero  InputSameDT=on  OutDataTypeStr=Inherit: Same as first input
  Relational Operator : RelationalOperator  Operator=<=  InputSameDT=on
  Relational Operator1 : RelationalOperator  Operator=<  InputSameDT=on
  Relational Operator2 : RelationalOperator  Operator=<=  InputSameDT=on
  Sum : Sum  Inputs=+++  AccumDataTypeStr=double  OutDataTypeStr=double  SaturateOnIntegerOverflow=on  InputSameDT=on
  Switch Case : SwitchCase  CaseConditions={1 2 3}
  input : Constant  Value=0.433
  input1 : Constant  Value=0.75
  input2 : Constant  Value=1.0
  Fex : Outport
  wires:
  Ve/1 -> Fcn/1
  Fcn/1 -> Product/2
  Ifd/1 -> Product/1
  Product/1 -> Gain/1
  Gain/1 -> Relational Operator2/1, 0.433<In<0.75/1(In), 0.75<=In<=1.0/1(In), In<=0.433/1(In), Relational Operator1/1, Relational Operator/1  "In"
  Merge/1 -> Fex/1
  0.75<=In<=1.0/1(f(In)) -> Merge/1
  0.433<In<0.75/1(f(In)) -> Merge/2
  In>1.0/1(f(In)) -> Merge/4
  In<=0.433/1(f(In)) -> Merge/3
  input1/1 -> Relational Operator1/2
  input2/1 -> Relational Operator2/2
  Relational Operator1/1 -> Sum/2
  Relational Operator/1 -> Sum/1
  Relational Operator2/1 -> Sum/3
  Sum/1 -> Switch Case/1
  Switch Case/1 -> 0.75<=In<=1.0/Action
  Switch Case/2 -> 0.433<In<0.75/Action
  Switch Case/3 -> In<=0.433/Action
  Switch Case/4 -> In>1.0/Action
  input/1 -> Relational Operator/2

== system power_machines_Hatch/EXCITATION1/AC1A/AC1A/Model/Continuous/Saturation Vx=Ve*Se[Ve] ==
  Ve : Inport
  Product : Product  SaturateOnIntegerOverflow=on  RndMeth=Zero  InputSameDT=on  OutDataTypeStr=Inherit: Same as first input
  Saturation : Lookup  InputValues=[0 Ve2 Ve1]  Table=[0 SeVe2 SeVe1]  SaturateOnIntegerOverflow=on
  Vx : Outport
  wires:
  Ve/1 -> Product/1, Saturation/1
  Saturation/1 -> Product/2
  Product/1 -> Vx/1

== system power_machines_Hatch/EXCITATION1/AC1A/AC1A/Model/Continuous/Transient Gain Reduction (Tc.s+1)//(Tb.s+1) ==
  In1 : Inport
  State Space : StateSpace  A=A  B=B  C=C  D=Dd  X0=X0
  Out1 : Outport  InitialOutput=0
  wires:
  State Space/1 -> Out1/1
  In1/1 -> State Space/1
